simulink model "nl3x2"  (Simulink 2.20)
settings: Solver=ode45  StartTime=0.0  StopTime=10.0  RelTol=1e-3
settings Model: ConsistencyChecking=off  RTWPlaceOutputsASAP=off  RTWLocalBlockOutputs=on  ExtModeTrigMode=oneshot

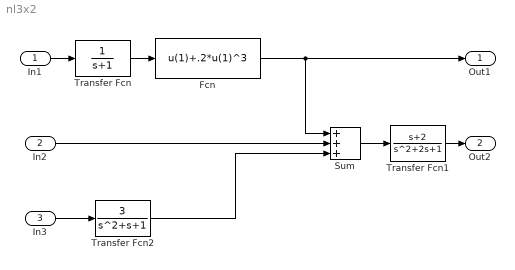
== system nl3x2 ==
  In1 : Inport  Port=1  PortWidth=-1  SampleTime=-1
  In2 : Inport  Port=2  PortWidth=-1  SampleTime=-1
  In3 : Inport  Port=3  PortWidth=-1  SampleTime=-1
  Fcn : Fcn  Expr=u(1)+.2*u(1)^3
  Sum : Sum  Inputs=+++
  Transfer Fcn : TransferFcn  Numerator=[1]  Denominator=[1 1]
  Transfer Fcn1 : TransferFcn  Numerator=[1 2]  Denominator=[1 2 1]
  Transfer Fcn2 : TransferFcn  Numerator=[3]  Denominator=[1 1 1]
  Out1 : Outport  Port=1
  Out2 : Outport  Port=2
  wires:
  In1/1 -> Transfer Fcn/1
  In3/1 -> Transfer Fcn2/1
  Transfer Fcn2/1 -> Sum/3
  Transfer Fcn/1 -> Fcn/1
  Fcn/1 -> Out1/1, Sum/1
  In2/1 -> Sum/2
  Transfer Fcn1/1 -> Out2/1
  Sum/1 -> Transfer Fcn1/1
